simulink model "GUI_User_V1_3"  (Simulink 7.7)
settings: Solver=FixedStepDiscrete  SolverMode=SingleTasking  StartTime=0.0  StopTime=60*60*24*365  FixedStep=0.001  RelTol=1e-3
InitFcn:
  | ADB=0;
  | p=1;
  | i1=0;
  | d=0.01;
  | filD=10;
  | 
  | SamT=0.001;
undefined symbols (not defined in the file or in its folder): kdc, tau
libraries: simulink x12, xpclib x2, Stewart_Gough_LibraryV2 x2
settings Model: Creator=LAB_Mecatronica_16  LastModifiedBy=Sebastian  SimulationMode=external  BufferReuse=off
settings DataIOCC: LimitDataPoints=off
settings OptimizationCC: BlockReduction=off  OptimizeBlockIOStorage=off  BufferReuse=off  ExpressionFolding=off  LocalBlockOutputs=off
settings HardwareCC: ProdIntDivRoundTo=Zero  ProdEndianess=LittleEndian  ProdHWDeviceType=Generic->32-bit x86 compatible
settings RTWCC: SystemTargetFile=xpctarget.tlc  TemplateMakefile=xpc_default_tmf  Description=xPC Target  ProcessScript=xpctarget_make_rtw_hook  RTWCompilerOptimization=On
settings xpcTargetCC: TargetFcnLib=ansi_tfl_table_tmw.mat  TargetFunctionLibrary=XPC_BLAS  FunctionExecutionProfile=off  CodeExecutionProfiling=off  ERTCodeCoverageTool=None  ParMdlRefBuildCompliant=on  CombineSignalStateStructs=off  PortableWordSizes=off  xPCTaskExecutionProfile=off  xPCRL32EventNumber=5000  xPCLoadParamSetFile=off  xPCConcurrentTasks=off  xPCEnableSFAnimation=off

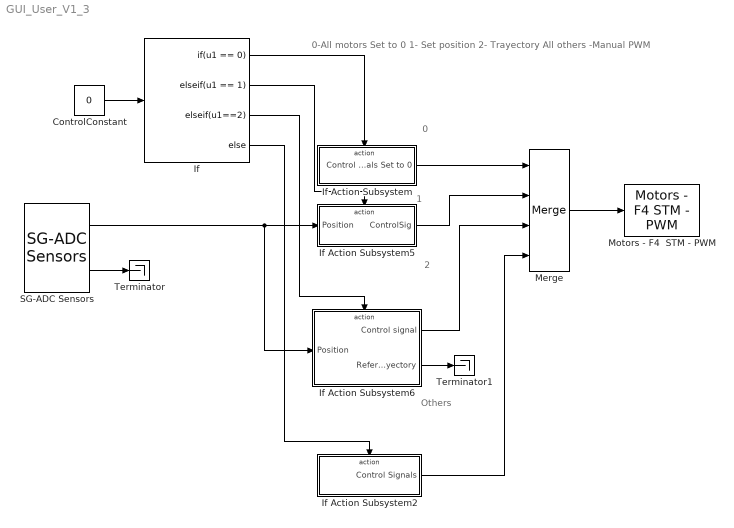
== system GUI_User_V1_3 ==
  note: 0-All motors Set to 0
      | 1- Set position
      | 2- Trayectory
      | All others -Manual PWM
  note: 0
  note: 1
  note: 2
  note: Others
  ControlConstant : Constant  Value=0
  If : If  IfExpression=u1 == 0  ElseIfExpressions=u1 == 1,u1==2
  If Action Subsystem : Subsystem  TreatAsAtomicUnit=on
  If Action Subsystem2 : Subsystem  TreatAsAtomicUnit=on
  If Action Subsystem5 : Subsystem  TreatAsAtomicUnit=on
  If Action Subsystem6 : Subsystem  TreatAsAtomicUnit=on
  Merge : Merge  Inputs=4  InitialOutput=[0 0 0 0 0 0]
  Motors - F4  STM - PWM : Stewart_Gough_LibraryV2/SG - Input//Output/Motors - F4  STM - PWM  SystemSampleTime=-1  Satura=80  SamTime=0.001
  SG-ADC Sensors : Stewart_Gough_LibraryV2/SG - Input//Output/SG-ADC Sensors  SystemSampleTime=-1  CutFreq=20  IniSt=[0 0 0 0 0 0]  SamTimeADC=0.001
  Terminator : Terminator
  Terminator1 : Terminator
  wires:
  ControlConstant/1 -> If/1
  SG-ADC Sensors/2 -> Terminator/1
  Merge/1 -> Motors - F4  STM - PWM/1
  If/1 -> If Action Subsystem/Action
  If Action Subsystem/1(Control Signals Set to 0) -> Merge/1
  SG-ADC Sensors/1 -> If Action Subsystem5/1(Position), If Action Subsystem6/1(Position)
  If/2 -> If Action Subsystem5/Action
  If/3 -> If Action Subsystem6/Action
  If/4 -> If Action Subsystem2/Action
  If Action Subsystem5/1(ControlSig) -> Merge/2
  If Action Subsystem6/1(Control signal) -> Merge/3
  If Action Subsystem2/1(Control Signals) -> Merge/4
  If Action Subsystem6/2(ReferenceTrayectory) -> Terminator1/1

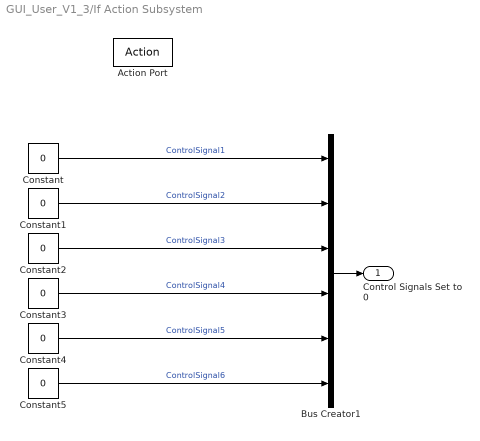
== system GUI_User_V1_3/If Action Subsystem ==
  Action Port : ActionPort  ActionType=then
  Bus Creator1 : BusCreator  Inputs=6
  Constant{,1..5} (6 alike) : Constant  Value=0
  Control Signals Set to 0 : Outport  InitialOutput=[0 0 0 0 0 0]
  wires:
  Constant/1 -> Bus Creator1/1  "ControlSignal1"
  Bus Creator1/1 -> Control Signals Set to 0/1
  Constant2/1 -> Bus Creator1/3  "ControlSignal3"
  Constant3/1 -> Bus Creator1/4  "ControlSignal4"
  Constant4/1 -> Bus Creator1/5  "ControlSignal5"
  Constant5/1 -> Bus Creator1/6  "ControlSignal6"
  Constant1/1 -> Bus Creator1/2  "ControlSignal2"

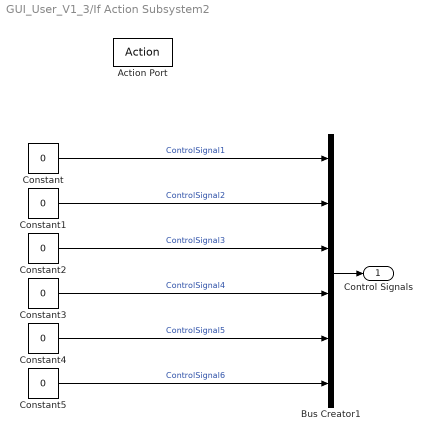
== system GUI_User_V1_3/If Action Subsystem2 ==
  Action Port : ActionPort  ActionType=else
  Bus Creator1 : BusCreator  Inputs=6
  Constant{,1..5} (6 alike) : Constant  Value=0
  Control Signals : Outport  InitialOutput=[0 0 0 0 0 0]
  wires:
  Constant/1 -> Bus Creator1/1  "ControlSignal1"
  Bus Creator1/1 -> Control Signals/1
  Constant2/1 -> Bus Creator1/3  "ControlSignal3"
  Constant3/1 -> Bus Creator1/4  "ControlSignal4"
  Constant4/1 -> Bus Creator1/5  "ControlSignal5"
  Constant5/1 -> Bus Creator1/6  "ControlSignal6"
  Constant1/1 -> Bus Creator1/2  "ControlSignal2"

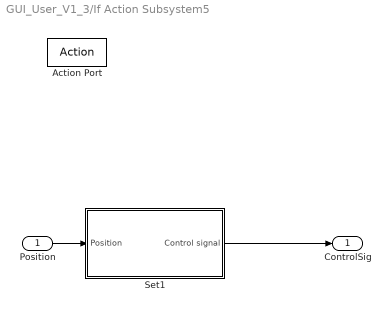
== system GUI_User_V1_3/If Action Subsystem5 ==
  Position : Inport
  Action Port : ActionPort  ActionType=elseif
  Set1 : Subsystem  mask(Set SG actuators to specific values){ActLen=[68.317      68.3214      68.3123      68.3123      68.3214       68.317], P1=2, I1=0, D1=0, Pole1=1, SamTime1=0.001}
      mask prompts: ActLen "Actuators length:"; P1 "P:"; I1 "I:"; D1 "D:"; Pole1 "Filter derivator (Hz):"; SamTime1 "Sample Time:"
      mask help: Set SG actuators to specific values through feedforward-PID controller
      mask init:
      | Pole2=1/(Pole1*2*pi);
      | tau(1)=12.9;
      | tau(2)=20.9;
      | tau(3)=16;
      | tau(4)=26.2;
      | tau(5)=17.1;
      | tau(6)=15.2;
      | kdc(1)=35.737;
      | kdc(2)=65.089;
      | kdc(3)=51.966;
      | kdc(4)=74.788;
      | kdc(5)=49.788;
      | kdc(6)=51.427;
  ControlSig : Outport  InitialOutput=[0 0 0 0 0 0]
  wires:
  Set1/1(Control signal) -> ControlSig/1
  Position/1 -> Set1/1(Position)

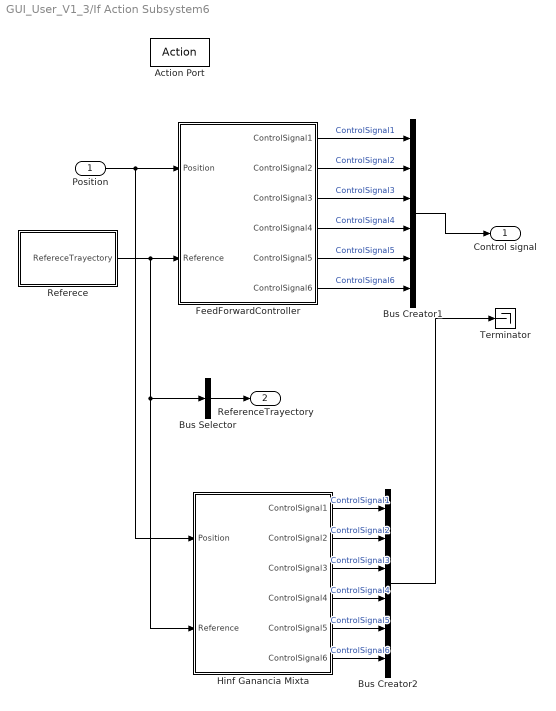
== system GUI_User_V1_3/If Action Subsystem6 ==
  Position : Inport
  Action Port : ActionPort  ActionType=elseif
  Bus Creator1 : BusCreator  Inputs=6
  Bus Creator2 : BusCreator  Inputs=6
  Bus Selector : BusSelector  OutputSignals=Position_1,Position_2,Position_3,Position_4,Position_5,Position_6,Velocity_1,Velocity_2,Velocity_3,Velocity_4,Velocity_5,Velocity_6  OutputAsBus=on
  FeedForwardController : Subsystem  mask(Feed forward controller for a stewart gough platform){Pff=2.5, Iff=2, Dff=0.1, DFff=10, SamTimeff=0.001}
      mask prompts: Pff "P"; Iff "I"; Dff "D"; DFff "Derivative Filter, Cutoff freq (Hz)"; SamTimeff "Sample Time"
      mask init:
      | DFff=1/(DFff*pi*2);
  Hinf Ganancia Mixta : Subsystem
  Referece : Subsystem
  Terminator : Terminator
  Control signal : Outport  InitialOutput=[0 0 0 0 0 0]
  ReferenceTrayectory : Outport  Port=2  InitialOutput=[0 0 0 0 0 0 0 0 0 0 0 0]
  wires:
  Position/1 -> FeedForwardController/1(Position), Hinf Ganancia Mixta/1(Position)
  Referece/1(RefereceTrayectory) -> FeedForwardController/2(Reference), Hinf Ganancia Mixta/2(Reference), Bus Selector/1
  FeedForwardController/1(ControlSignal1) -> Bus Creator1/1  "ControlSignal1"
  FeedForwardController/2(ControlSignal2) -> Bus Creator1/2  "ControlSignal2"
  FeedForwardController/3(ControlSignal3) -> Bus Creator1/3  "ControlSignal3"
  FeedForwardController/4(ControlSignal4) -> Bus Creator1/4  "ControlSignal4"
  FeedForwardController/5(ControlSignal5) -> Bus Creator1/5  "ControlSignal5"
  FeedForwardController/6(ControlSignal6) -> Bus Creator1/6  "ControlSignal6"
  Hinf Ganancia Mixta/1(ControlSignal1) -> Bus Creator2/1  "ControlSignal1"
  Hinf Ganancia Mixta/2(ControlSignal2) -> Bus Creator2/2  "ControlSignal2"
  Hinf Ganancia Mixta/3(ControlSignal3) -> Bus Creator2/3  "ControlSignal3"
  Hinf Ganancia Mixta/4(ControlSignal4) -> Bus Creator2/4  "ControlSignal4"
  Hinf Ganancia Mixta/5(ControlSignal5) -> Bus Creator2/5  "ControlSignal5"
  Hinf Ganancia Mixta/6(ControlSignal6) -> Bus Creator2/6  "ControlSignal6"
  Bus Selector/1 -> ReferenceTrayectory/1
  Bus Creator1/1 -> Control signal/1
  Bus Creator2/1 -> Terminator/1

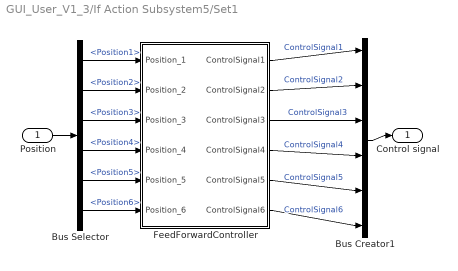
== system GUI_User_V1_3/If Action Subsystem5/Set1 ==
  Position : Inport
  Bus Creator1 : BusCreator  Inputs=6
  Bus Selector : BusSelector  OutputSignals=Position1,Position2,Position3,Position4,Position5,Position6
  FeedForwardController : Subsystem
  Control signal : Outport
  wires:
  Bus Selector/1 -> FeedForwardController/1(Position_1)  "<Position1>"
  Bus Selector/2 -> FeedForwardController/2(Position_2)  "<Position2>"
  Bus Selector/3 -> FeedForwardController/3(Position_3)  "<Position3>"
  Bus Selector/4 -> FeedForwardController/4(Position_4)  "<Position4>"
  Bus Selector/5 -> FeedForwardController/5(Position_5)  "<Position5>"
  Bus Selector/6 -> FeedForwardController/6(Position_6)  "<Position6>"
  FeedForwardController/1(ControlSignal1) -> Bus Creator1/1  "ControlSignal1"
  FeedForwardController/2(ControlSignal2) -> Bus Creator1/2  "ControlSignal2"
  FeedForwardController/3(ControlSignal3) -> Bus Creator1/3  "ControlSignal3"
  FeedForwardController/4(ControlSignal4) -> Bus Creator1/4  "ControlSignal4"
  FeedForwardController/5(ControlSignal5) -> Bus Creator1/5  "ControlSignal5"
  FeedForwardController/6(ControlSignal6) -> Bus Creator1/6  "ControlSignal6"
  Bus Creator1/1 -> Control signal/1
  Position/1 -> Bus Selector/1

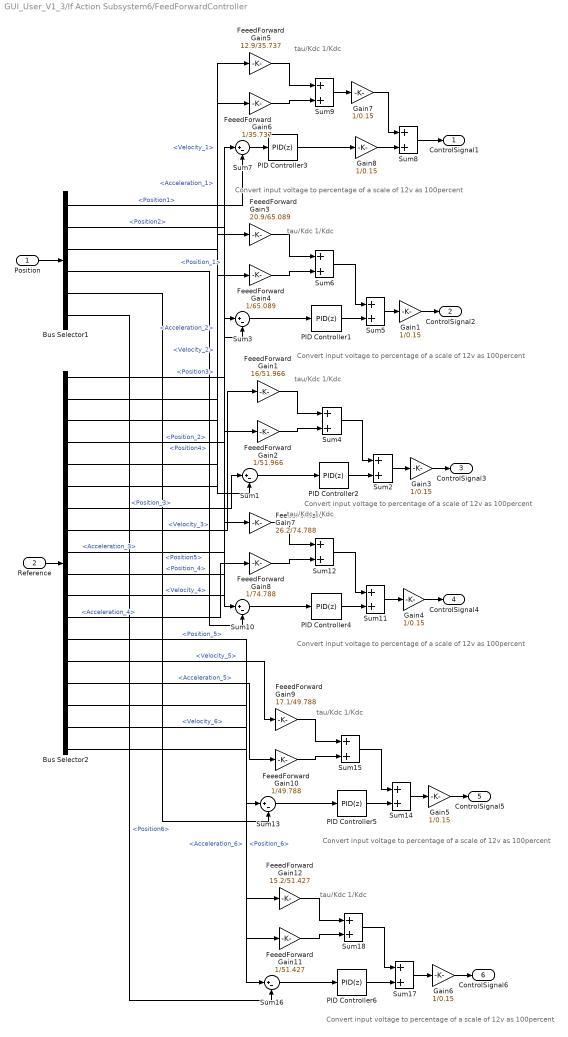
== system GUI_User_V1_3/If Action Subsystem6/FeedForwardController ==
  note: Convert input voltage
      |  to percentage  of a
      | scale of 12v as
      | 100percent
  note: Convert input voltage
      |  to percentage  of a
      | scale of 12v as
      | 100percent
  note: Convert input voltage
      |  to percentage  of a
      | scale of 12v as
      | 100percent
  note: Convert input voltage
      |  to percentage  of a
      | scale of 12v as
      | 100percent
  note: Convert input voltage
      |  to percentage  of a
      | scale of 12v as
      | 100percent
  note: Convert input voltage
      |  to percentage  of a
      | scale of 12v as
      | 100percent
  note: tau/Kdc
      | 1/Kdc
  note: tau/Kdc
      | 1/Kdc
  note: tau/Kdc
      | 1/Kdc
  note: tau/Kdc
      | 1/Kdc
  note: tau/Kdc
      | 1/Kdc
  note: tau/Kdc
      | 1/Kdc
  Position : Inport
  Reference : Inport  Port=2
  Bus Selector1 : BusSelector  OutputSignals=Position1,Position2,Position3,Position4,Position5,Position6
  Bus Selector2 : BusSelector  OutputSignals=Position_1,Velocity_1,Acceleration_1,Position_2,Velocity_2,Acceleration_2,Position_3,Velocity_3,Acceleration_3,Position_4,Velocity_4,Acceleration_4,Position_5,Velocity_5,Acceleration_5,Position_6,Velocity_6,Acceleration_6
  FeeedForward Gain1 : Gain  Gain=16/51.966
  FeeedForward Gain10 : Gain  Gain=1/49.788
  FeeedForward Gain11 : Gain  Gain=1/51.427
  FeeedForward Gain12 : Gain  Gain=15.2/51.427
  FeeedForward Gain2 : Gain  Gain=1/51.966
  FeeedForward Gain3 : Gain  Gain=20.9/65.089
  FeeedForward Gain4 : Gain  Gain=1/65.089
  FeeedForward Gain5 : Gain  Gain=12.9/35.737
  FeeedForward Gain6 : Gain  Gain=1/35.737
  FeeedForward Gain7 : Gain  Gain=26.2/74.788
  FeeedForward Gain8 : Gain  Gain=1/74.788
  FeeedForward Gain9 : Gain  Gain=17.1/49.788
  Gain{1,3..8} (7 alike) : Gain  Gain=1/0.15
  PID Controller{1..6} (6 alike) : simulink/Continuous/PID Controller  SystemSampleTime=-1  Controller=PID  TimeDomain=Discrete-time  SampleTime=SamTimeff  IntegratorMethod=Forward Euler  FilterMethod=Forward Euler  Form=Parallel  P=Pff  I=Iff  D=Dff  N=DFff  InitialConditionSource=internal  InitialConditionForIntegrator=0  InitialConditionForFilter=0  ExternalReset=none  LimitOutput=off  UpperSaturationLimit=inf  LowerSaturationLimit=-inf  LinearizeAsGain=off  AntiWindupMode=none  Kb=1  TrackingMode=off  Kt=1  PParamMin=[]  PParamMax=[]  IParamMin=[]  IParamMax=[]  DParamMin=[]  DParamMax=[]  NParamMin=[]  NParamMax=[]  KbParamMin=[]  KbParamMax=[]  KtParamMin=[]  KtParamMax=[]  POutMin=[]  POutMax=[]  IOutMin=[]  IOutMax=[]  DOutMin=[]  DOutMax=[]  NOutMin=[]  NOutMax=[]  KbOutMin=[]  KbOutMax=[]  KtOutMin=[]  KtOutMax=[]  IntegratorOutMin=[]  IntegratorOutMax=[]  FilterOutMin=[]  FilterOutMax=[]  SumOutMin=[]  SumOutMax=[]  SumI1OutMin=[]  SumI1OutMax=[]  SumI2OutMin=[]  SumI2OutMax=[]  SumI3OutMin=[]  SumI3OutMax=[]  SumDOutMin=[]  SumDOutMax=[]  SaturationOutMin=[]  SaturationOutMax=[]  IntegratorContinuousStateAttributes=''  IntegratorStateMustResolveToSignalObject=off  IntegratorRTWStateStorageClass=Auto  FilterContinuousStateAttributes=''  FilterStateMustResolveToSignalObject=off  FilterRTWStateStorageClass=Auto
  Sum{1,3,7,10,13,16} (6 alike) : Sum  Inputs=|+-
  Sum{2,4..6,8..9,11..12,14..15,17..18} (12 alike) : Sum
  ControlSignal1 : Outport
  ControlSignal2 : Outport  Port=2
  ControlSignal3 : Outport  Port=3
  ControlSignal4 : Outport  Port=4
  ControlSignal5 : Outport  Port=5
  ControlSignal6 : Outport  Port=6
  wires:
  Gain7/1 -> Sum8/1
  Sum9/1 -> Gain7/1
  Gain8/1 -> Sum8/2
  PID Controller3/1 -> Gain8/1
  FeeedForward Gain2/1 -> Sum4/2
  FeeedForward Gain1/1 -> Sum4/1
  Sum4/1 -> Sum2/1
  Sum2/1 -> Gain3/1
  Sum1/1 -> PID Controller2/1
  PID Controller2/1 -> Sum2/2
  FeeedForward Gain4/1 -> Sum6/2
  FeeedForward Gain3/1 -> Sum6/1
  Sum6/1 -> Sum5/1
  Sum5/1 -> Gain1/1
  Sum3/1 -> PID Controller1/1
  PID Controller1/1 -> Sum5/2
  FeeedForward Gain6/1 -> Sum9/2
  FeeedForward Gain5/1 -> Sum9/1
  Sum7/1 -> PID Controller3/1
  FeeedForward Gain8/1 -> Sum12/2
  FeeedForward Gain7/1 -> Sum12/1
  Sum12/1 -> Sum11/1
  Sum11/1 -> Gain4/1
  Sum10/1 -> PID Controller4/1
  PID Controller4/1 -> Sum11/2
  FeeedForward Gain10/1 -> Sum15/2
  FeeedForward Gain9/1 -> Sum15/1
  Sum15/1 -> Sum14/1
  Sum14/1 -> Gain5/1
  Sum13/1 -> PID Controller5/1
  PID Controller5/1 -> Sum14/2
  FeeedForward Gain11/1 -> Sum18/2
  FeeedForward Gain12/1 -> Sum18/1
  Sum18/1 -> Sum17/1
  Sum17/1 -> Gain6/1
  Sum16/1 -> PID Controller6/1
  PID Controller6/1 -> Sum17/2
  Bus Selector1/1 -> Sum7/2  "<Position1>"
  Bus Selector1/2 -> Sum3/2  "<Position2>"
  Bus Selector1/3 -> Sum1/2  "<Position3>"
  Bus Selector1/4 -> Sum10/2  "<Position4>"
  Bus Selector1/5 -> Sum13/2  "<Position5>"
  Bus Selector1/6 -> Sum16/2  "<Position6>"
  Bus Selector2/1 -> Sum7/1  "<Position_1>"
  Bus Selector2/2 -> FeeedForward Gain5/1  "<Velocity_1>"
  Bus Selector2/3 -> FeeedForward Gain6/1  "<Acceleration_1>"
  Bus Selector2/4 -> Sum3/1  "<Position_2>"
  Bus Selector2/5 -> FeeedForward Gain3/1  "<Velocity_2>"
  Bus Selector2/6 -> FeeedForward Gain4/1  "<Acceleration_2>"
  Bus Selector2/7 -> Sum1/1  "<Position_3>"
  Bus Selector2/8 -> FeeedForward Gain1/1  "<Velocity_3>"
  Bus Selector2/9 -> FeeedForward Gain2/1  "<Acceleration_3>"
  Bus Selector2/10 -> Sum10/1  "<Position_4>"
  Bus Selector2/11 -> FeeedForward Gain7/1  "<Velocity_4>"
  Bus Selector2/12 -> FeeedForward Gain8/1  "<Acceleration_4>"
  Bus Selector2/13 -> Sum13/1  "<Position_5>"
  Bus Selector2/14 -> FeeedForward Gain9/1  "<Velocity_5>"
  Bus Selector2/15 -> FeeedForward Gain10/1  "<Acceleration_5>"
  Bus Selector2/16 -> Sum16/1  "<Position_6>"
  Bus Selector2/17 -> FeeedForward Gain12/1  "<Velocity_6>"
  Bus Selector2/18 -> FeeedForward Gain11/1  "<Acceleration_6>"
  Position/1 -> Bus Selector1/1
  Sum8/1 -> ControlSignal1/1
  Gain1/1 -> ControlSignal2/1
  Gain3/1 -> ControlSignal3/1
  Reference/1 -> Bus Selector2/1
  Gain4/1 -> ControlSignal4/1
  Gain5/1 -> ControlSignal5/1
  Gain6/1 -> ControlSignal6/1

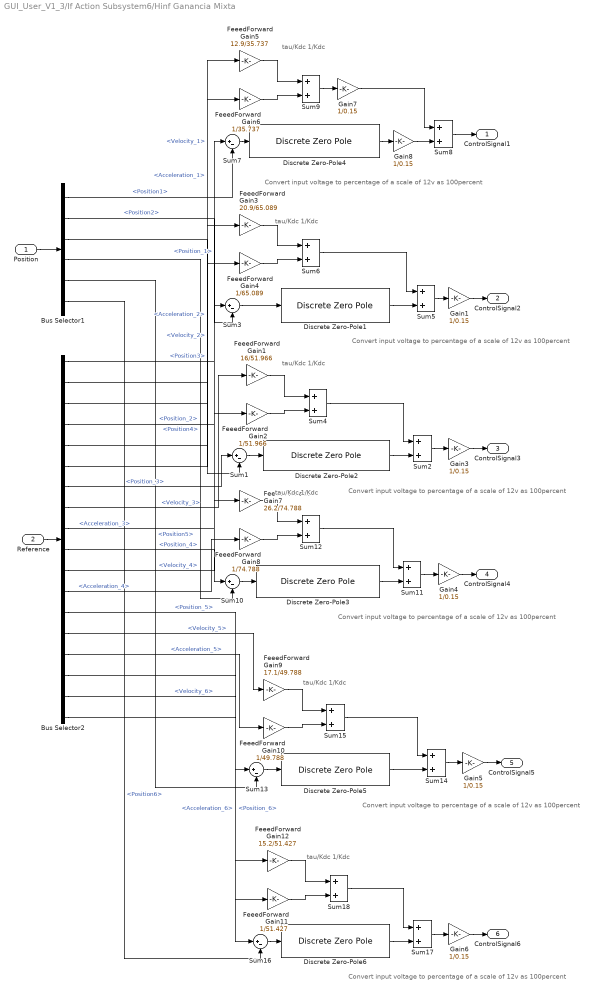
== system GUI_User_V1_3/If Action Subsystem6/Hinf Ganancia Mixta ==
  note: Convert input voltage
      |  to percentage  of a
      | scale of 12v as
      | 100percent
  note: Convert input voltage
      |  to percentage  of a
      | scale of 12v as
      | 100percent
  note: Convert input voltage
      |  to percentage  of a
      | scale of 12v as
      | 100percent
  note: Convert input voltage
      |  to percentage  of a
      | scale of 12v as
      | 100percent
  note: Convert input voltage
      |  to percentage  of a
      | scale of 12v as
      | 100percent
  note: Convert input voltage
      |  to percentage  of a
      | scale of 12v as
      | 100percent
  note: tau/Kdc
      | 1/Kdc
  note: tau/Kdc
      | 1/Kdc
  note: tau/Kdc
      | 1/Kdc
  note: tau/Kdc
      | 1/Kdc
  note: tau/Kdc
      | 1/Kdc
  note: tau/Kdc
      | 1/Kdc
  Position : Inport
  Reference : Inport  Port=2
  Bus Selector1 : BusSelector  OutputSignals=Position1,Position2,Position3,Position4,Position5,Position6
  Bus Selector2 : BusSelector  OutputSignals=Position_1,Velocity_1,Acceleration_1,Position_2,Velocity_2,Acceleration_2,Position_3,Velocity_3,Acceleration_3,Position_4,Velocity_4,Acceleration_4,Position_5,Velocity_5,Acceleration_5,Position_6,Velocity_6,Acceleration_6
  Discrete Zero-Pole1 : DiscreteZeroPole  Zeros=[0.07914 0.9792 1]  Poles=[0.08506 0.6115 0.8444 1]  Gain=2.9617  SampleTime=0.001
  Discrete Zero-Pole2 : DiscreteZeroPole  Zeros=[1 0.984 0.07978]  Poles=[0.08352 0.6783 0.831 1]  Gain=3.3372  SampleTime=0.001
  Discrete Zero-Pole3 : DiscreteZeroPole  Zeros=[1 0.974 0.0786]  Poles=[0.08649 0.5657 0.8495 1]  Gain=2.7876  SampleTime=0.001
  Discrete Zero-Pole4 : DiscreteZeroPole  Zeros=[1 0.9871 0.08041]  Poles=[0.08216 1 0.7872 0.7688]  Gain=4.4402  SampleTime=0.001
  Discrete Zero-Pole5 : DiscreteZeroPole  Zeros=[1 0.983 0.07988]  Poles=[0.0833 0.69 0.8258 1]  Gain=3.4633  SampleTime=0.001
  Discrete Zero-Pole6 : DiscreteZeroPole  Zeros=[1 0.9848 0.07981]  Poles=[0.08346 0.6812 0.8308 1]  Gain=3.3456  SampleTime=0.001
  FeeedForward Gain1 : Gain  Gain=16/51.966
  FeeedForward Gain10 : Gain  Gain=1/49.788
  FeeedForward Gain11 : Gain  Gain=1/51.427
  FeeedForward Gain12 : Gain  Gain=15.2/51.427
  FeeedForward Gain2 : Gain  Gain=1/51.966
  FeeedForward Gain3 : Gain  Gain=20.9/65.089
  FeeedForward Gain4 : Gain  Gain=1/65.089
  FeeedForward Gain5 : Gain  Gain=12.9/35.737
  FeeedForward Gain6 : Gain  Gain=1/35.737
  FeeedForward Gain7 : Gain  Gain=26.2/74.788
  FeeedForward Gain8 : Gain  Gain=1/74.788
  FeeedForward Gain9 : Gain  Gain=17.1/49.788
  Gain{1,3..8} (7 alike) : Gain  Gain=1/0.15
  Sum{1,3,7,10,13,16} (6 alike) : Sum  Inputs=|+-
  Sum{2,4..6,8..9,11..12,14..15,17..18} (12 alike) : Sum
  ControlSignal1 : Outport
  ControlSignal2 : Outport  Port=2
  ControlSignal3 : Outport  Port=3
  ControlSignal4 : Outport  Port=4
  ControlSignal5 : Outport  Port=5
  ControlSignal6 : Outport  Port=6
  wires:
  Gain7/1 -> Sum8/1
  Sum9/1 -> Gain7/1
  Gain8/1 -> Sum8/2
  FeeedForward Gain2/1 -> Sum4/2
  FeeedForward Gain1/1 -> Sum4/1
  Sum4/1 -> Sum2/1
  Sum2/1 -> Gain3/1
  Discrete Zero-Pole2/1 -> Sum2/2
  FeeedForward Gain4/1 -> Sum6/2
  FeeedForward Gain3/1 -> Sum6/1
  Sum6/1 -> Sum5/1
  Sum5/1 -> Gain1/1
  Sum3/1 -> Discrete Zero-Pole1/1
  Discrete Zero-Pole1/1 -> Sum5/2
  FeeedForward Gain6/1 -> Sum9/2
  FeeedForward Gain5/1 -> Sum9/1
  Sum7/1 -> Discrete Zero-Pole4/1
  FeeedForward Gain8/1 -> Sum12/2
  FeeedForward Gain7/1 -> Sum12/1
  Sum12/1 -> Sum11/1
  Sum11/1 -> Gain4/1
  FeeedForward Gain10/1 -> Sum15/2
  FeeedForward Gain9/1 -> Sum15/1
  Sum15/1 -> Sum14/1
  Sum14/1 -> Gain5/1
  FeeedForward Gain11/1 -> Sum18/2
  FeeedForward Gain12/1 -> Sum18/1
  Sum18/1 -> Sum17/1
  Sum17/1 -> Gain6/1
  Bus Selector1/1 -> Sum7/2  "<Position1>"
  Bus Selector1/2 -> Sum3/2  "<Position2>"
  Bus Selector1/3 -> Sum1/2  "<Position3>"
  Bus Selector1/4 -> Sum10/2  "<Position4>"
  Bus Selector1/5 -> Sum13/2  "<Position5>"
  Bus Selector1/6 -> Sum16/2  "<Position6>"
  Bus Selector2/1 -> Sum7/1  "<Position_1>"
  Bus Selector2/2 -> FeeedForward Gain5/1  "<Velocity_1>"
  Bus Selector2/3 -> FeeedForward Gain6/1  "<Acceleration_1>"
  Bus Selector2/4 -> Sum3/1  "<Position_2>"
  Bus Selector2/5 -> FeeedForward Gain3/1  "<Velocity_2>"
  Bus Selector2/6 -> FeeedForward Gain4/1  "<Acceleration_2>"
  Bus Selector2/7 -> Sum1/1  "<Position_3>"
  Bus Selector2/8 -> FeeedForward Gain1/1  "<Velocity_3>"
  Bus Selector2/9 -> FeeedForward Gain2/1  "<Acceleration_3>"
  Bus Selector2/10 -> Sum10/1  "<Position_4>"
  Bus Selector2/11 -> FeeedForward Gain7/1  "<Velocity_4>"
  Bus Selector2/12 -> FeeedForward Gain8/1  "<Acceleration_4>"
  Bus Selector2/13 -> Sum13/1  "<Position_5>"
  Bus Selector2/14 -> FeeedForward Gain9/1  "<Velocity_5>"
  Bus Selector2/15 -> FeeedForward Gain10/1  "<Acceleration_5>"
  Bus Selector2/16 -> Sum16/1  "<Position_6>"
  Bus Selector2/17 -> FeeedForward Gain12/1  "<Velocity_6>"
  Bus Selector2/18 -> FeeedForward Gain11/1  "<Acceleration_6>"
  Position/1 -> Bus Selector1/1
  Sum8/1 -> ControlSignal1/1
  Gain1/1 -> ControlSignal2/1
  Gain3/1 -> ControlSignal3/1
  Reference/1 -> Bus Selector2/1
  Gain4/1 -> ControlSignal4/1
  Gain5/1 -> ControlSignal5/1
  Gain6/1 -> ControlSignal6/1
  Discrete Zero-Pole4/1 -> Gain8/1
  Sum1/1 -> Discrete Zero-Pole2/1
  Sum10/1 -> Discrete Zero-Pole3/1
  Discrete Zero-Pole3/1 -> Sum11/2
  Sum13/1 -> Discrete Zero-Pole5/1
  Discrete Zero-Pole5/1 -> Sum14/2
  Sum16/1 -> Discrete Zero-Pole6/1
  Discrete Zero-Pole6/1 -> Sum17/2

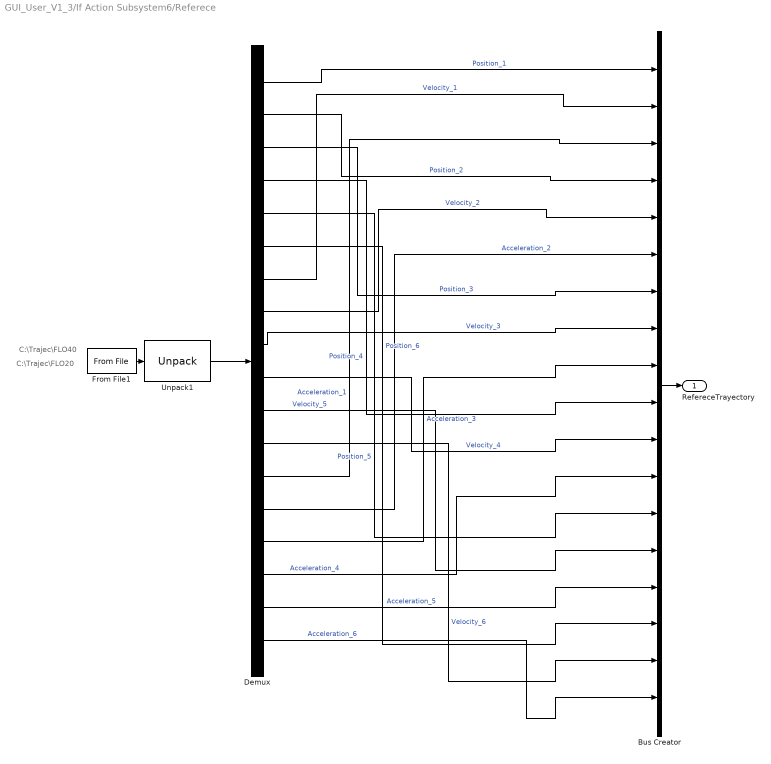
== system GUI_User_V1_3/If Action Subsystem6/Referece ==
  note: C:\Trajec\FLO40
  note: C:\Trajec\FLO20
  Bus Creator : BusCreator  Inputs=18
  Demux : Demux  Outputs=18
  From File1 : xpclib/Misc./From File  filename='C:\xpcfiles\Trajec2.dat'  dataSize=8*18  bufSize=40000*18*20  readSize=512  EOFOption=Hold last output  sampTime=0.001
  Unpack1 : xpclib/UDP/Unpack  dimensions={[18]}  datatypes={'double'}  byteAlign=1
  RefereceTrayectory : Outport
  wires:
  Demux/1 -> Bus Creator/1  "Position_1"
  Demux/7 -> Bus Creator/2  "Velocity_1"
  Demux/13 -> Bus Creator/3  "Acceleration_1"
  Demux/2 -> Bus Creator/4  "Position_2"
  Demux/8 -> Bus Creator/5  "Velocity_2"
  Demux/14 -> Bus Creator/6  "Acceleration_2"
  Demux/3 -> Bus Creator/7  "Position_3"
  Demux/9 -> Bus Creator/8  "Velocity_3"
  Demux/15 -> Bus Creator/9  "Acceleration_3"
  Demux/4 -> Bus Creator/10  "Position_4"
  Demux/10 -> Bus Creator/11  "Velocity_4"
  Demux/16 -> Bus Creator/12  "Acceleration_4"
  Demux/5 -> Bus Creator/13  "Position_5"
  Demux/11 -> Bus Creator/14  "Velocity_5"
  Demux/17 -> Bus Creator/15  "Acceleration_5"
  Demux/6 -> Bus Creator/16  "Position_6"
  Demux/12 -> Bus Creator/17  "Velocity_6"
  Demux/18 -> Bus Creator/18  "Acceleration_6"
  Bus Creator/1 -> RefereceTrayectory/1
  From File1/1 -> Unpack1/1
  Unpack1/1 -> Demux/1

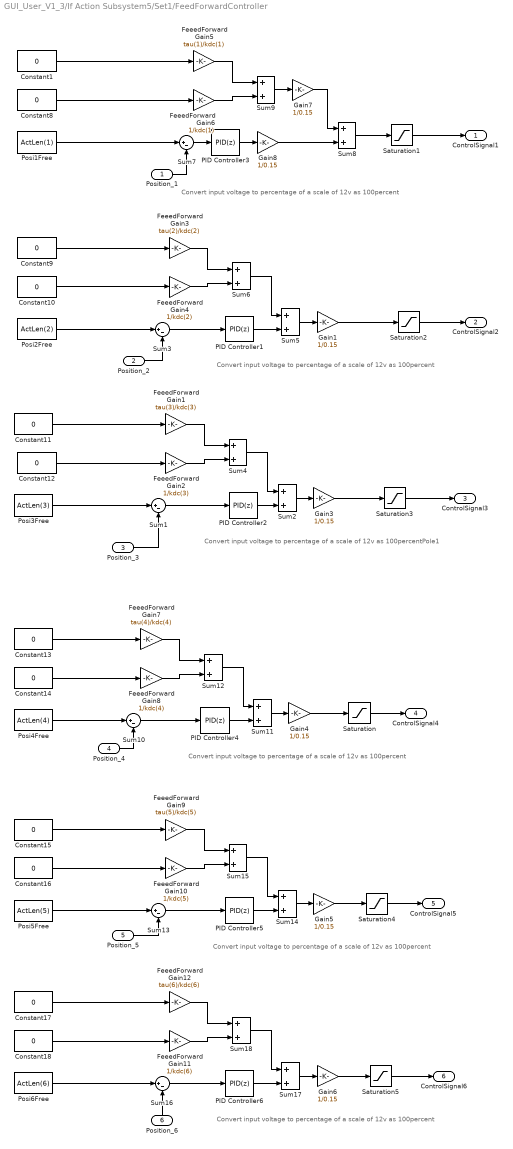
== system GUI_User_V1_3/If Action Subsystem5/Set1/FeedForwardController ==
  note: Convert input voltage
      |  to percentage  of a
      | scale of 12v as
      | 100percent
  note: Convert input voltage
      |  to percentage  of a
      | scale of 12v as
      | 100percent
  note: Convert input voltage
      |  to percentage  of a
      | scale of 12v as
      | 100percent
  note: Convert input voltage
      |  to percentage  of a
      | scale of 12v as
      | 100percent
  note: Convert input voltage
      |  to percentage  of a
      | scale of 12v as
      | 100percent
  note: Convert input voltage
      |  to percentage  of a
      | scale of 12v as
      | 100percentPole1
  Position_1 : Inport
  Position_2 : Inport  Port=2
  Position_3 : Inport  Port=3
  Position_4 : Inport  Port=4
  Position_5 : Inport  Port=5
  Position_6 : Inport  Port=6
  Constant{1,8..18} (12 alike) : Constant  Value=0
  FeeedForward Gain1 : Gain  Gain=tau(3)/kdc(3)
  FeeedForward Gain10 : Gain  Gain=1/kdc(5)
  FeeedForward Gain11 : Gain  Gain=1/kdc(6)
  FeeedForward Gain12 : Gain  Gain=tau(6)/kdc(6)
  FeeedForward Gain2 : Gain  Gain=1/kdc(3)
  FeeedForward Gain3 : Gain  Gain=tau(2)/kdc(2)
  FeeedForward Gain4 : Gain  Gain=1/kdc(2)
  FeeedForward Gain5 : Gain  Gain=tau(1)/kdc(1)
  FeeedForward Gain6 : Gain  Gain=1/kdc(1)
  FeeedForward Gain7 : Gain  Gain=tau(4)/kdc(4)
  FeeedForward Gain8 : Gain  Gain=1/kdc(4)
  FeeedForward Gain9 : Gain  Gain=tau(5)/kdc(5)
  Gain{1,3..8} (7 alike) : Gain  Gain=1/0.15
  PID Controller{1..6} (6 alike) : simulink/Continuous/PID Controller  SystemSampleTime=-1  Controller=PID  TimeDomain=Discrete-time  SampleTime=SamTime1  IntegratorMethod=Forward Euler  FilterMethod=Forward Euler  Form=Parallel  P=P1  I=I1  D=D1  N=Pole2  InitialConditionSource=internal  InitialConditionForIntegrator=0  InitialConditionForFilter=0  ExternalReset=none  LimitOutput=off  UpperSaturationLimit=inf  LowerSaturationLimit=-inf  LinearizeAsGain=off  AntiWindupMode=none  Kb=1  TrackingMode=off  Kt=1  PParamMin=[]  PParamMax=[]  IParamMin=[]  IParamMax=[]  DParamMin=[]  DParamMax=[]  NParamMin=[]  NParamMax=[]  KbParamMin=[]  KbParamMax=[]  KtParamMin=[]  KtParamMax=[]  POutMin=[]  POutMax=[]  IOutMin=[]  IOutMax=[]  DOutMin=[]  DOutMax=[]  NOutMin=[]  NOutMax=[]  KbOutMin=[]  KbOutMax=[]  KtOutMin=[]  KtOutMax=[]  IntegratorOutMin=[]  IntegratorOutMax=[]  FilterOutMin=[]  FilterOutMax=[]  SumOutMin=[]  SumOutMax=[]  SumI1OutMin=[]  SumI1OutMax=[]  SumI2OutMin=[]  SumI2OutMax=[]  SumI3OutMin=[]  SumI3OutMax=[]  SumDOutMin=[]  SumDOutMax=[]  SaturationOutMin=[]  SaturationOutMax=[]  IntegratorContinuousStateAttributes=''  IntegratorStateMustResolveToSignalObject=off  IntegratorRTWStateStorageClass=Auto  FilterContinuousStateAttributes=''  FilterStateMustResolveToSignalObject=off  FilterRTWStateStorageClass=Auto
  Posi1Free : Constant  Value=ActLen(1)
  Posi2Free : Constant  Value=ActLen(2)
  Posi3Free : Constant  Value=ActLen(3)
  Posi4Free : Constant  Value=ActLen(4)
  Posi5Free : Constant  Value=ActLen(5)
  Posi6Free : Constant  Value=ActLen(6)
  Saturation{,1..5} (6 alike) : Saturate  UpperLimit=40  LowerLimit=-40
  Sum{1,3,7,10,13,16} (6 alike) : Sum  Inputs=|+-
  Sum{2,4..6,8..9,11..12,14..15,17..18} (12 alike) : Sum
  ControlSignal1 : Outport
  ControlSignal2 : Outport  Port=2
  ControlSignal3 : Outport  Port=3
  ControlSignal4 : Outport  Port=4
  ControlSignal5 : Outport  Port=5
  ControlSignal6 : Outport  Port=6
  wires:
  Posi5Free/1 -> Sum13/1
  Constant16/1 -> FeeedForward Gain10/1
  Constant15/1 -> FeeedForward Gain9/1
  Posi6Free/1 -> Sum16/1
  Constant18/1 -> FeeedForward Gain11/1
  Posi3Free/1 -> Sum1/1
  Constant12/1 -> FeeedForward Gain2/1
  Constant13/1 -> FeeedForward Gain7/1
  Constant14/1 -> FeeedForward Gain8/1
  Posi4Free/1 -> Sum10/1
  Constant11/1 -> FeeedForward Gain1/1
  Posi2Free/1 -> Sum3/1
  Constant10/1 -> FeeedForward Gain4/1
  Constant9/1 -> FeeedForward Gain3/1
  Posi1Free/1 -> Sum7/1
  Constant8/1 -> FeeedForward Gain6/1
  Constant1/1 -> FeeedForward Gain5/1
  PID Controller6/1 -> Sum17/2
  Sum16/1 -> PID Controller6/1
  Sum17/1 -> Gain6/1
  Sum18/1 -> Sum17/1
  FeeedForward Gain12/1 -> Sum18/1
  FeeedForward Gain11/1 -> Sum18/2
  PID Controller5/1 -> Sum14/2
  Sum13/1 -> PID Controller5/1
  Sum14/1 -> Gain5/1
  Sum15/1 -> Sum14/1
  FeeedForward Gain9/1 -> Sum15/1
  FeeedForward Gain10/1 -> Sum15/2
  PID Controller4/1 -> Sum11/2
  Sum10/1 -> PID Controller4/1
  Sum11/1 -> Gain4/1
  Sum12/1 -> Sum11/1
  FeeedForward Gain7/1 -> Sum12/1
  FeeedForward Gain8/1 -> Sum12/2
  Sum7/1 -> PID Controller3/1
  Sum8/1 -> Saturation1/1
  FeeedForward Gain5/1 -> Sum9/1
  FeeedForward Gain6/1 -> Sum9/2
  PID Controller1/1 -> Sum5/2
  Sum3/1 -> PID Controller1/1
  Sum5/1 -> Gain1/1
  Sum6/1 -> Sum5/1
  FeeedForward Gain3/1 -> Sum6/1
  FeeedForward Gain4/1 -> Sum6/2
  PID Controller2/1 -> Sum2/2
  Sum1/1 -> PID Controller2/1
  Sum2/1 -> Gain3/1
  Sum4/1 -> Sum2/1
  FeeedForward Gain1/1 -> Sum4/1
  FeeedForward Gain2/1 -> Sum4/2
  Position_6/1 -> Sum16/2
  Position_1/1 -> Sum7/2
  Position_2/1 -> Sum3/2
  Position_3/1 -> Sum1/2
  Position_4/1 -> Sum10/2
  Position_5/1 -> Sum13/2
  PID Controller3/1 -> Gain8/1
  Gain8/1 -> Sum8/2
  Sum9/1 -> Gain7/1
  Gain7/1 -> Sum8/1
  Constant17/1 -> FeeedForward Gain12/1
  Gain1/1 -> Saturation2/1
  Gain3/1 -> Saturation3/1
  Gain4/1 -> Saturation/1
  Gain5/1 -> Saturation4/1
  Gain6/1 -> Saturation5/1
  Saturation/1 -> ControlSignal4/1
  Saturation1/1 -> ControlSignal1/1
  Saturation2/1 -> ControlSignal2/1
  Saturation3/1 -> ControlSignal3/1
  Saturation4/1 -> ControlSignal5/1
  Saturation5/1 -> ControlSignal6/1
